simulink model "Project_3_model"  (R2023b)
settings: Solver=VariableStepAuto  StartTime=0.0  StopTime=10.0  RelTol=1e-3
values from neighbouring files (symbols this model uses):
  C0 = 0.0041    [init.m]
  C1 = 0.000066    (= 6.6e-05)    [init.m]
  C2 = 0.5*Rho*A*Cd    (= 0.51156)    [init.m]
  M = 1000    [init.m]
settings Model: Creator=danie  LastModifiedBy=danie

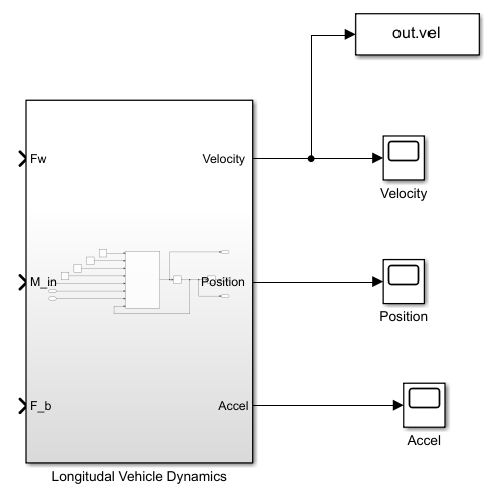
[thumbnail: Simulink's stored preview of the top-level diagram]
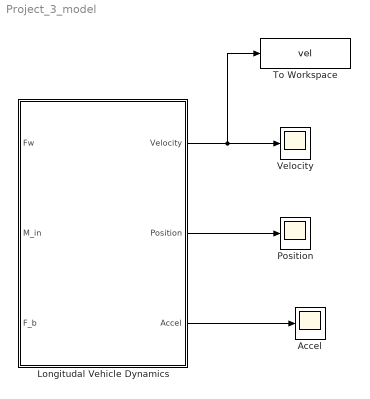
== system Project_3_model ==
  Accel : Scope
  Longitudal Vehicle Dynamics : Subsystem
  Position : Scope
  To Workspace : ToWorkspace  VariableName=vel  SaveFormat=Timeseries  SampleTime=-1
  Velocity : Scope
  wires:
  Longitudal Vehicle Dynamics/1("Velocity ") -> To Workspace/1, Velocity/1
  Longitudal Vehicle Dynamics/2("Position ") -> Position/1
  Longitudal Vehicle Dynamics/3(Accel) -> Accel/1

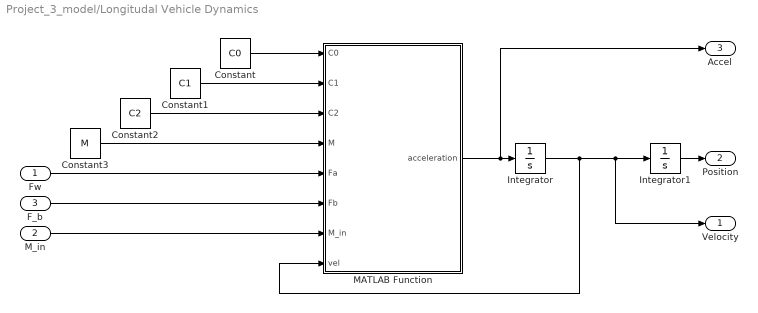
== system Project_3_model/Longitudal Vehicle Dynamics ==
  "Fw " : Inport
  "M_in " : Inport  Port=2
  "F_b " : Inport  Port=3
  Constant : Constant  Value=C0
  Constant1 : Constant  Value=C1
  Constant2 : Constant  Value=C2
  Constant3 : Constant  Value=M
  Integrator : Integrator  LimitOutput=on  LowerSaturationLimit=0
  Integrator1 : Integrator
  MATLAB Function : MATLAB Function  TreatAsAtomicUnit=on
  "Velocity " : Outport  VectorParamsAs1DForOutWhenUnconnected=off
  "Position " : Outport  Port=2  VectorParamsAs1DForOutWhenUnconnected=off
  Accel : Outport  Port=3
  wires:
  Constant1/1 -> MATLAB Function/2(C1)
  Constant/1 -> MATLAB Function/1(C0)
  MATLAB Function/1(acceleration) -> Accel/1, Integrator/1
  Constant2/1 -> MATLAB Function/3(C2)
  Constant3/1 -> MATLAB Function/4(M)
  "Fw "/1 -> MATLAB Function/5(Fa)
  "F_b "/1 -> MATLAB Function/6(Fb)
  Integrator/1 -> MATLAB Function/8(vel), "Velocity "/1, Integrator1/1
  Integrator1/1 -> "Position "/1
  "M_in "/1 -> MATLAB Function/7(M_in)

== matlab function Project_3_model/Longitudal Vehicle Dynamics/MATLAB Function ==
  data: C0 input; acceleration output; C1 input; C2 input; M input; Fa input; Fb input; M_in input; vel input
function acceleration   = vehicle(C0,C1,C2,M,Fa,Fb,M_in, vel)

acceleration = (((Fa-Fb))-(C0+ C1*vel + C2*(vel)^2))/(M+M_in);
